simulink model "regulador_niveis"  (R2022b)
settings: Solver=VariableStepAuto  StartTime=0.0  StopTime=10.0  RelTol=1e-3
values from neighbouring files (symbols this model uses):
  A1 = planta.tanque_1.A    [obterMalhaTanque.m]    (also in obterMalhaTanque1.m; projetarControladorAnalitico.m; projetarControladorTanque1Analitico.m; projetarControladorTunando.m)
  A2 = planta.tanque_2.A    [obterMalhaTanque.m]    (also in obterMalhaTanque2.m; projetarControladorAnalitico.m; projetarControladorTanque2Analitico.m; projetarControladorTunando.m)
  controlador = obterControlador(tipo_de_projeto, '"iter"')    [plotarProjeto.m]    (also in plotarProjetoAnalitico.m = projetarControladorTunando(requisitos, planta); plotarProjetoNelderMead.m = obterControladorNelderMead(requisitos, planta); plotarSimulacao.m = projetarControladorPSO(requisitos,planta, display_mode); projetarControladorTanque1NelderMead.m = projetarControladorNelderMeadGenerico(requisitos.tanque_1, p)
  R1 = planta.R1    [obterMalhaTanque.m]    (also in obterMalhaTanque1.m; obterMalhaTanque2.m; projetarControladorAnalitico.m; projetarControladorTanque1Analitico.m)
  R2 = planta.R2    [obterMalhaTanque.m]    (also in obterMalhaTanque2.m; projetarControladorAnalitico.m; projetarControladorTanque2Analitico.m; projetarControladorTunando.m)
libraries: slpidlib x1
settings Model: Creator=Beato  LastModifiedBy=Beato

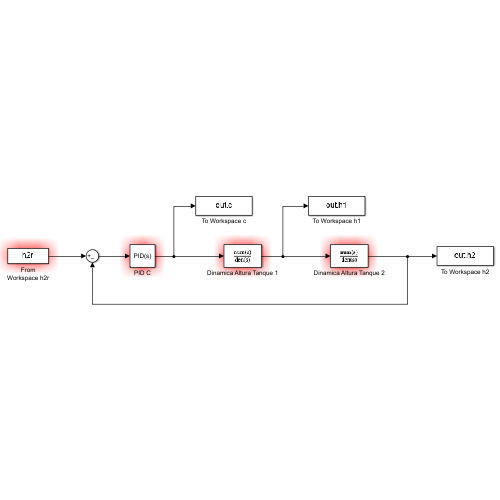
[thumbnail: Simulink's stored preview of the top-level diagram]
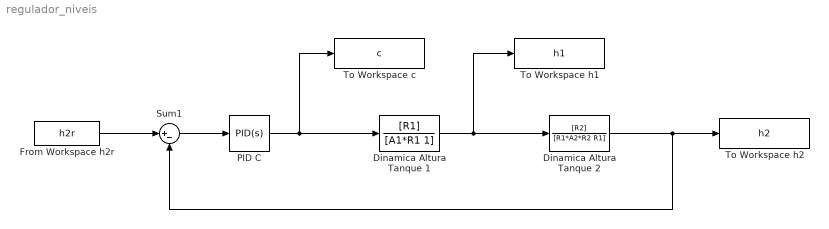
== system regulador_niveis ==
  Dinamica Altura Tanque 1 : TransferFcn  Numerator=[R1]  Denominator=[A1*R1 1]
  Dinamica Altura Tanque 2 : TransferFcn  Numerator=[R2]  Denominator=[R1*A2*R2 R1]
  From Workspace h2r : FromWorkspace  VariableName=h2r
  PID C : slpidlib/PID Controller  Controller=PID  Form=Parallel  TimeDomain=Continuous-time  UseExternalTs=off  SampleTime=-1  IntegratorMethod=Forward Euler  FilterMethod=Forward Euler  ControllerParametersSource=internal  P=controlador.Kp  I=controlador.Ki  UseKiTs=off  D=controlador.Kd  N=100  UseFilter=on  TunerSelectOption=Transfer Function Based (PID Tuner App)  InitialConditionSource=internal  InitialConditionForIntegrator=0  InitialConditionForFilter=0  DifferentiatorICPrevScaledInput=0  ExternalReset=none  TrackingMode=off  Kt=1  LimitOutput=off  SatLimitsSource=internal  UpperSaturationLimit=inf  LowerSaturationLimit=-inf  LinearizeAsGain=on  AntiWindupMode=none  Kb=1  LimitIntegrator=off  UpperIntegratorSaturationLimit=inf  LowerIntegratorSaturationLimit=-inf  POutMin=[]  POutMax=[]  IOutMin=[]  IOutMax=[]  DOutMin=[]  DOutMax=[]  NOutMin=[]  NOutMax=[]  SumOutMin=[]  SumOutMax=[]  SaturationOutMin=[]  SaturationOutMax=[]  PParamMin=[]  PParamMax=[]  IParamMin=[]  IParamMax=[]  DParamMin=[]  DParamMax=[]  NParamMin=[]  NParamMax=[]  KbParamMin=[]  KbParamMax=[]  KtParamMin=[]  KtParamMax=[]  KbOutMin=[]  KbOutMax=[]  KtOutMin=[]  KtOutMax=[]  IntegratorOutMin=[]  IntegratorOutMax=[]  FilterOutMin=[]  FilterOutMax=[]  SumI1OutMin=[]  SumI1OutMax=[]  SumI2OutMin=[]  SumI2OutMax=[]  SumI3OutMin=[]  SumI3OutMax=[]  SumI4OutMin=[]  SumI4OutMax=[]  SumDOutMin=[]  SumDOutMax=[]  DifferentiatorOutMin=[]  DifferentiatorOutMax=[]  FilterDiffOutCoefMin=[]  FilterDiffOutCoefMax=[]  ReciprocalOutMin=[]  ReciprocalOutMax=[]  SumDenOutMin=[]  SumDenOutMax=[]  SumNumOutMin=[]  SumNumOutMax=[]  DivideOutMin=[]  DivideOutMax=[]  UdiffTsProdOutMin=[]  UdiffTsProdOutMax=[]  NTsProdOutMin=[]  NTsProdOutMax=[]  UintegralTsProdOutMin=[]  UintegralTsProdOutMax=[]  UngainTsProdOutMin=[]  UngainTsProdOutMax=[]  ClampingZeroOutDataTypeStr=Inherit: Inherit via back propagation  ClampingZeroOutMin=[]  ClampingZeroOutMax=[]  FilterDenConstantOutDataTypeStr=Inherit: Inherit via back propagation  FilterDenConstantOutMin=[]  FilterDenConstantOutMax=[]  PCopyOutDataTypeStr=Inherit: Inherit via back propagation  PCopyOutMin=[]  PCopyOutMax=[]  NCopyOutDataTypeStr=Inherit: Inherit via back propagation  NCopyOutMin=[]  NCopyOutMax=[]  IntegratorContinuousStateAttributes=''  IntegratorStateMustResolveToSignalObject=off  IntegratorRTWStateStorageClass=Auto  FilterContinuousStateAttributes=''  FilterStateMustResolveToSignalObject=off  FilterRTWStateStorageClass=Auto  ParallelPVariant=InternalParameters  IdealPVariant=Disabled  IVariant=InternalParameters  DVariant=InternalParameters  IntegratorVariant=Continuous  SatVariant=Disabled  AWVariant=Passthrough  PCopyVariant=Disabled  TRVariant=Disabled  FdbkBlocksVariant=Forward  IdealPFdbkVariant=Disabled  SatFdbkVariant=Disabled  DerivativeFilterVariant=ContFilter  NVariant=InternalParameters  NCopyVariant=Disabled  FilterICVariant=InternalICsFilter  IntegratorICVariant=InternalICs  ExternalResetVariant=Disabled  TRSumVariant=Passthrough  SumFdbkVariant=Disabled  SumVariant=Sum_PID  TsampFilterVariant=InternalTs  TsampNgainVariant=Passthrough  TsampIntegralVariant=Passthrough  ExternalSaturationOutDataTypeStr=Inherit: Same as second input
  Sum1 : Sum  Inputs=|+-
  To Workspace c : ToWorkspace  VariableName=c  SaveFormat=Timeseries  SampleTime=-1
  To Workspace h1 : ToWorkspace  VariableName=h1  SaveFormat=Timeseries  SampleTime=-1
  To Workspace h2 : ToWorkspace  VariableName=h2  SaveFormat=Timeseries  SampleTime=-1
  wires:
  PID C/1 -> Dinamica Altura Tanque 1/1, To Workspace c/1
  Sum1/1 -> PID C/1
  From Workspace h2r/1 -> Sum1/1
  Dinamica Altura Tanque 2/1 -> To Workspace h2/1, Sum1/2
  Dinamica Altura Tanque 1/1 -> Dinamica Altura Tanque 2/1, To Workspace h1/1
